simulink model "vrtut1"  (Simulink 6.0)
settings: Solver=ode45  StartTime=0.0  StopTime=100  RelTol=1e-3
libraries: simulink x3, vrlib x2
settings Model: CovMetricSettings=d  Creator=Straka  LastModifiedBy=Houska  ExtModeTrigMode=oneshot  ExtModeArmWhenConnect=off
settings DataIOCC: LimitDataPoints=off  SignalLoggingName=logsOut
settings OptimizationCC: BlockReduction=off  BooleanDataType=off
settings DebuggingCC: CheckExecutionContextPreStartOutputMsg=on  CheckExecutionContextRuntimeOutputMsg=on  SolverPrmCheckMsg=none
settings HardwareCC: TargetUnknown=on
settings ModelReferenceCC: UpdateModelReferenceTargets=IfOutOfDate
settings GRTTargetCC: LifeSpan=inf
settings SFSimCC: SFSimApplyToAllLibs=on  SFSimBuildMode=Incremental

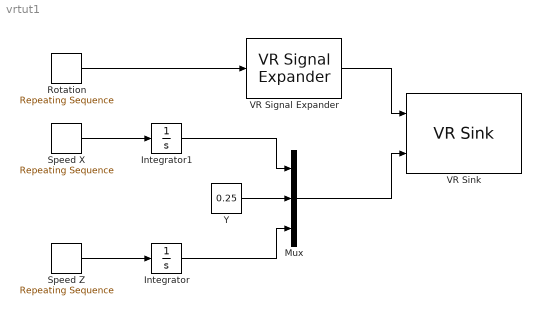
== system vrtut1 ==
  Integrator : Integrator  UpperSaturationLimit=Inf  LowerSaturationLimit=-Inf  ZeroCross=off
  Integrator1 : Integrator  InitialCondition=3  UpperSaturationLimit=Inf  LowerSaturationLimit=-Inf  ZeroCross=off
  Mux : Mux  Inputs=3
  Rotation : simulink/Sources/Repeating Sequence  rep_seq_t=[0 20 22 80 82 100]  rep_seq_y=[-1.57 -1.57 -0.7 -0.7 0 0]
  Speed X : simulink/Sources/Repeating Sequence  rep_seq_t=[0 20 22 80 82 100]  rep_seq_y=[0 0 0.33 0.33 0.7 0.7]
  Speed Z : simulink/Sources/Repeating Sequence  rep_seq_t=[0 20 22 80 82 100]  rep_seq_y=[0.55 0.55 0.24 0.24 0 0]
  VR Signal Expander : vrlib/VR Signal Expander  outwidth=4  outidx=4
  VR Sink : vrlib/VR Sink  SampleTime=0.2  ViewEnable=on  RemoteChange=off  RemoteView=off  FieldsWritten=Automobile.rotation.4.1.double#Automobile.translation.3.1.double  WorldFileName=vrmount.wrl  AutoView=on
  Y : Constant  Value=0.25
  wires:
  Speed X/1 -> Integrator1/1
  Speed Z/1 -> Integrator/1
  Y/1 -> Mux/2
  Integrator1/1 -> Mux/1
  Integrator/1 -> Mux/3
  Mux/1 -> VR Sink/2
  VR Signal Expander/1 -> VR Sink/1
  Rotation/1 -> VR Signal Expander/1
